simulink model "E"  (R2019a)
settings: Solver=VariableStepAuto  StartTime=0.0  StopTime=25  RelTol=1e-3
values from neighbouring files (symbols this model uses):
  A = sys_d.a    [ss2dt.m]    (also in vars.m = [[ 0.      0.      1.      0.    ])
  B = sys_d.b    [ss2dt.m]    (also in vars.m = [[0.        ])
  C = sys_d.c    [ss2dt.m]    (also in vars.m = [[1. 0. 0. 0.])
  K = [[ -2.00366979 199.78340569  -6.64587178  52.07504646]]    [vars.m]
  L = [[ 2.45    0.15  ] ... (first row only)    [vars.m]
settings Model: Creator=Artem  LastModifiedBy=Artem

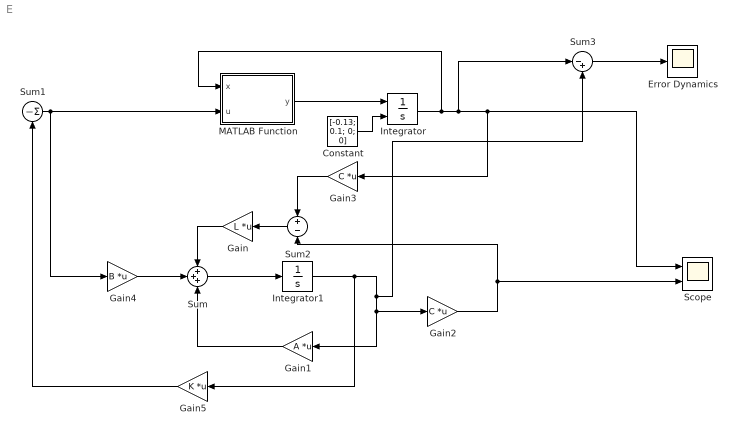
== system E ==
  Constant : Constant  Value=[-0.13; 0.1; 0; 0]
  "Error Dynamics " : Scope
  Gain : Gain  Gain=L  Multiplication=Matrix(K*u)
  Gain1 : Gain  Gain=A  Multiplication=Matrix(K*u)
  Gain2 : Gain  Gain=C  Multiplication=Matrix(K*u)
  Gain3 : Gain  Gain=C  Multiplication=Matrix(K*u)
  Gain4 : Gain  Gain=B  Multiplication=Matrix(K*u)
  Gain5 : Gain  Gain=K  Multiplication=Matrix(K*u)
  Integrator : Integrator  InitialConditionSource=external
  Integrator1 : Integrator
  MATLAB Function : MATLAB Function  TreatAsAtomicUnit=on
  Scope : Scope  NumInputPorts=2
  Sum : Sum  Inputs=+++
  Sum1 : Sum  Inputs=||-
  Sum2 : Sum  Inputs=+-
  Sum3 : Sum  Inputs=|-+
  wires:
  Gain5/1 -> Sum1/1
  Gain1/1 -> Sum/3
  Gain3/1 -> Sum2/1
  Gain/1 -> Sum/1
  Sum2/1 -> Gain/1
  Sum1/1 -> Gain4/1, MATLAB Function/2(u)
  Sum3/1 -> "Error Dynamics "/1
  Integrator1/1 -> Gain5/1, Sum3/2, Gain2/1, Gain1/1
  Integrator/1 -> Gain3/1, Scope/1, Sum3/1, MATLAB Function/1(x)
  Gain2/1 -> Scope/2, Sum2/2
  Sum/1 -> Integrator1/1
  Constant/1 -> Integrator/2
  MATLAB Function/1(y) -> Integrator/1
  Gain4/1 -> Sum/2

== matlab function E/MATLAB Function ==
  data: x input; u input; y output
function y = fcn(x,u)
g = 9.8;
m = 4.4;
M = 7.5;
l = 1.2;

x2 = @(theta,theta_, F) (m * sin(theta) * (g * cos(theta)  - l * theta_ ^ 2) + F) / (M + m * sin(theta) ^ 2);
theta2 = @(theta,theta_, F) ((g * (M+m)-l*m*cos(theta)*theta_^2 )* sin(theta) + F * cos(theta))/ (l * (M + m * sin(theta)^2));

y = [x(3);
     x(4);
     x2(x(2),x(4),u);
     theta2(x(2),x(4),u)];
